simulink model "cp_simulink_model"  (R2020a)
settings: Solver=VariableStepAuto  StartTime=0.0  StopTime=6  RelTol=1e-3
model workspace (MAT data in the model file):
  K = [-2050.38878007 -370.974368426 -90.1104778242 -925.652821526]
  fr = [3.42970671828 53.6033015773]
  par = [0.188 0.07 0.04165 0.0035 0.0201 29.1 0.0538 9.81 0.15 100 0.005]
settings Model: EnablePacing=on  Creator=antal  LastModifiedBy=antal

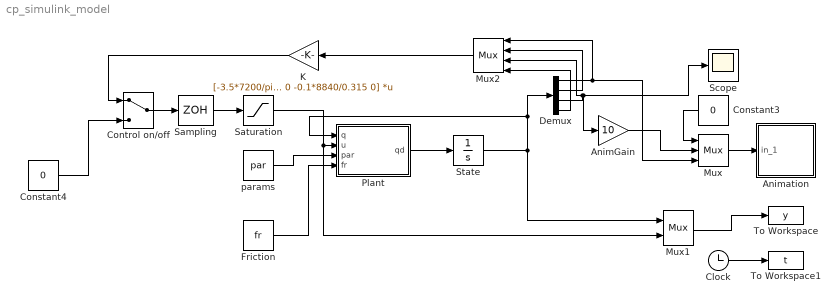
== system cp_simulink_model ==
  AnimGain : Gain  Gain=10
  Animation : Subsystem  mask(Pendulum plot){RefBlock=Constant3}
      mask prompts: RefBlock "DC reference signal block name:"
      mask help: Pendulum plot
      mask Help: Pendulum animation function using Handle graphics.
      mask Display: plot([-10 10],[0 0],[-2 -2 2 2],[0 1 1 0],[0 3],[1 5])
  Clock : Clock
  Constant3 : Constant  Value=0
  Constant4 : Constant  Value=0
  Control on/off : ManualSwitch
  Demux : Demux
  Friction : Constant  Value=fr
  K : Gain  Gain=[-3.5*7200/pi 0 -0.1*8840/0.315 0]  Multiplication=Matrix(K*u)
  Mux : Mux  Inputs=3
  Mux1 : Mux  Inputs=2
  Mux2 : Mux
  Plant : MATLAB Function  TreatAsAtomicUnit=on
  Sampling : ZeroOrderHold  SampleTime=0.02
  Saturation : Saturate  UpperLimit=40  LowerLimit=-40
  Scope : Scope
  State : Integrator  InitialCondition=[0.1;0;0;0]
  To Workspace : ToWorkspace  VariableName=y  SampleTime=0.002
  To Workspace1 : ToWorkspace  VariableName=t  SampleTime=0.002
  params : Constant  Value=par  VectorParams1D=off
  wires:
  Demux/4 -> Mux2/4
  Mux2/1 -> K/1
  Clock/1 -> To Workspace1/1
  Control on/off/1 -> Sampling/1
  Constant4/1 -> Control on/off/2
  K/1 -> Control on/off/1
  Mux/1 -> Animation/1(in_1)
  params/1 -> Plant/3(par)
  Constant3/1 -> Mux/1
  Friction/1 -> Plant/4(fr)
  Mux1/1 -> To Workspace/1
  State/1 -> Plant/1(q), Demux/1, Mux1/1
  Plant/1(qd) -> State/1
  Demux/2 -> Mux2/2
  Demux/1 -> Mux2/1, Mux/3
  AnimGain/1 -> Mux/2
  Demux/3 -> Scope/1, AnimGain/1, Mux2/3
  Saturation/1 -> Plant/2(u), Mux1/2
  Sampling/1 -> Saturation/1

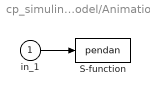
== system cp_simulink_model/Animation ==
  in_1 : Inport
  S-function : S-Function  FunctionName=pendan  Parameters=RefBlock  SFunctionDeploymentMode=off  EnableBusSupport=off
      settings: DeleteFcn=pendan([],[],[],'DeleteBlock');
  wires:
  in_1/1 -> S-function/1

== matlab function cp_simulink_model/Plant ==
  data: q input; u input; qd output; par input; fr input
function qd = fcn(q,u,par,fr)
qd = zeros(size(q));
phi = q(1);
phid = q(2);
x = q(3);
xd = q(4);
m = par(1); m_0 = par(2); k_m = par(3); R = par(4); L_a = par(5);
R_a = par(6); k_e = par(7); g = par(8); s = par(9);

qd(1,1) = phid;      % dphidt = dphidt

qd(2,1) = ((m+m_0)*g*sin(phi) - (k_m/R/R_a*(u-k_e/R*xd)-fr(1)*...
    tanh(xd*fr(2)))*cos(phi) -...
     m*s*phid^2*sin(phi)*cos(phi)) / (4/3*s*(m+m_0) - m*s*cos(phi)^2);

qd(3,1) = xd; 
 
qd(4,1) = (k_m/R/R_a*(u-k_e/R*xd)-fr(1)*tanh(xd*fr(2))- 3/4*m*g*sin(phi)*cos(phi) +...
    m*s*phid^2*sin(phi)) / (m+m_0-3/4*m*cos(phi)^2);
